simulink library "carnotUIBK"  (R2024b)
settings: Solver=VariableStepAuto  StartTime=0.0  StopTime=10.0  RelTol=1e-3  EnableMultiTasking=on
values from neighbouring files (symbols this model uses):
  area = area + room(kk).area    [THERMALZONE.m]
  boundary = BOUNDARY()    [BUILDING.m]
  building = obj    [BUILDING.m]
  C = zeros(1,length(d)+1)    [CONSTRUCTION.m]
  cp = str2num(value)    [CONSTRUCTION.m]
  pos = find(d_layer>0)    [CONSTRUCTION.m]
  rho = str2num(value)    [CONSTRUCTION.m]
  type = 1    [CONSTRUCTION.m]
  zone = obj.zone(ind)    [THERMALZONE.m]
undefined symbols (not defined in the file or in its folder): A, amb_factor, B, const, control, Dd, get_building, height, p, Qdot_C, Qdot_H, Qdot_I_electricity, Qdot_I_light, Qdot_I_person, Qdot_S, Qdot_T_ground, Qdot_T_neighbour, Qdot_T_opaque, Qdot_T_window, Qdot_V_infiltration, Qdot_V_mech, Qdot_V_window, r_frame, solar_ratio, solar_ratio1, solar_ratio2, Tc, Tr, Ts, Uvalue, view_factor, wall, wallsurface, window, window_height, window_heigth, window_width, windowsurface, x_CO2, x_H2O, x_VOC, z
libraries: carnot x105, $bdroot x22, simulink x18, simulink_extras x14
(part 4 of 13)

== system carnotUIBK/wall_intersection/EMPTY ==
  AIB1 : Inport
  AIB2 : Inport  Port=2
  Qdot_sol1 : Inport  Port=3
  Qdot_sol2 : Inport  Port=4
  Constant : Constant  Value=zeros(1,2)
  Constant1 : Constant  Value=zeros(1,5)
  Constant2 : Constant  Value=zeros(1,12)
  Constant3 : Constant  Value=zeros(1,2)
  Constant4 : Constant  Value=zeros(1,5)
  Constant5 : Constant  Value=zeros(1,12)
  Mux1 : Mux  Inputs=[2 5 12]
  Mux2 : Mux  Inputs=[2 5 12]
  Terminator{,2,4..5} (4 alike) : Terminator
  solar_ratio1 : Gain  Gain=solar_ratio1
  solar_ratio2 : Gain  Gain=solar_ratio2
  "[S1]" : Outport  VectorParamsAs1DForOutWhenUnconnected=off
  "[S2]" : Outport  Port=2  VectorParamsAs1DForOutWhenUnconnected=off
  wires:
  solar_ratio1/1 -> Terminator4/1
  Constant2/1 -> Mux1/3
  Qdot_sol1/1 -> solar_ratio1/1
  AIB1/1 -> Terminator2/1
  Constant/1 -> Mux1/1
  Mux1/1 -> "[S1]"/1
  Constant1/1 -> Mux1/2
  AIB2/1 -> Terminator/1
  solar_ratio2/1 -> Terminator5/1
  Qdot_sol2/1 -> solar_ratio2/1
  Constant5/1 -> Mux2/3
  Constant3/1 -> Mux2/1
  Mux2/1 -> "[S2]"/1
  Constant4/1 -> Mux2/2

== system carnotUIBK/wall_intersection/R-C model ==
  AIB1 : Inport
  AIB2 : Inport  Port=2
  Qdot_sol1 : Inport  Port=3
  Qdot_sol2 : Inport  Port=4
  Ground : Ground
  Terminator{,1..3,5} (5 alike) : Terminator
  Wall_basic1 : carnot/Basic/Thermal_Models/Wall_basic  tau=tau  t0=t0  d=d  dactive=dactive  cond=cond  cwall=cwall  rho=rho
      settings: SourceProductName=Carnot
  alpha_i1 : Subsystem  Variant=on  mask{view_factor=view_factor}
  alpha_i2 : Subsystem  Variant=on  mask{view_factor=amb_factor}
  nohygrothermal : Constant  Value=0
  solar_ratio1 : Gain  Gain=solar_ratio1
  solar_ratio2 : Gain  Gain=solar_ratio2
  "[S1]" : Outport  VectorParamsAs1DForOutWhenUnconnected=off
  "[S2]" : Outport  Port=2  VectorParamsAs1DForOutWhenUnconnected=off
  wires:
  alpha_i1/2("[S]") -> "[S1]"/1
  alpha_i1/3(alpha_c) -> Terminator/1
  nohygrothermal/1 -> alpha_i2/4(phis), alpha_i1/4(phis)
  solar_ratio1/1 -> alpha_i1/3(Qdot sol)
  Qdot_sol1/1 -> solar_ratio1/1
  alpha_i1/1(qdots) -> Wall_basic1/3
  alpha_i2/1(qdots) -> Wall_basic1/1
  Wall_basic1/3 -> alpha_i1/1(Ts)
  Wall_basic1/1 -> alpha_i2/1(Ts)
  Wall_basic1/2 -> Terminator5/1
  Ground/1 -> Wall_basic1/2
  Qdot_sol2/1 -> solar_ratio2/1
  AIB1/1 -> alpha_i1/2(AIB)
  AIB2/1 -> alpha_i2/2(AIB)
  solar_ratio2/1 -> alpha_i2/3(Qdot sol)
  alpha_i2/3(alpha_c) -> Terminator2/1
  alpha_i2/2("[S]") -> "[S2]"/1
  alpha_i1/4(phi_i_1/100) -> Terminator1/1
  alpha_i2/4(phi_i_1/100) -> Terminator3/1

== system carnotUIBK/wall_intersection/UA ==
  AIB1 : Inport
  AIB2 : Inport  Port=2
  Qdot_sol1 : Inport  Port=3
  Qdot_sol2 : Inport  Port=4
  1/U : Constant  Value=1/U
  Add : Sum  Inputs=2
  Add1 : Sum  Inputs=+-
  Bus Selector1 : BusSelector  OutputSignals=Ts
  Bus Selector2 : BusSelector  OutputSignals=Ts
  Constant1 : Constant  Value=zeros(1,9)
  Constant10 : Constant  Value=zeros(1,9)
  Constant2 : Constant  Value=zeros(1,7)
  Constant8 : Constant  Value=zeros(1,7)
  Gain : Gain  Gain=-1
  Mux1 : Mux  Inputs=[1 1 7 1 9]
  Mux4 : Mux  Inputs=[1 1 7 1 9]
  Qdot : Sum  Inputs=2
  Qdot1 : Sum  Inputs=2
  Qdot_T : Product  Inputs=**/
  Qdotr/Qdotc : Gain  Gain=0.5
  Qdotr/Qdotc1 : Gain  Gain=0.5
  Rsi : Subsystem  Variant=on
  solar_ratio1 : Gain  Gain=solar_ratio1
  solar_ratio2 : Gain  Gain=solar_ratio2
  wallsurface : Constant  Value=wallsurface
  "[S1]" : Outport  VectorParamsAs1DForOutWhenUnconnected=off
  "[S2]" : Outport  Port=2  VectorParamsAs1DForOutWhenUnconnected=off
  wires:
  Qdot_sol1/1 -> solar_ratio1/1
  Qdot_sol2/1 -> solar_ratio2/1
  Bus Selector1/1 -> Add1/2  "<Ts>"
  Add1/1 -> Qdot_T/1
  Add/1 -> Qdot_T/3
  wallsurface/1 -> Qdot_T/2
  Rsi/1(Rsi) -> Add/2
  1/U/1 -> Add/1
  AIB1/1 -> Bus Selector1/1
  AIB2/1 -> Bus Selector2/1
  Bus Selector2/1 -> Add1/1  "<Ts>"
  Mux4/1 -> "[S1]"/1
  Qdotr/Qdotc/1 -> Mux4/2, Mux4/1
  solar_ratio1/1 -> Qdot/2
  Mux1/1 -> "[S2]"/1
  Qdotr/Qdotc1/1 -> Mux1/2, Mux1/1
  Qdot1/1 -> Mux1/4, Qdotr/Qdotc1/1
  Gain/1 -> Qdot1/1
  solar_ratio2/1 -> Qdot1/2
  Constant10/1 -> Mux4/5
  Constant8/1 -> Mux4/3
  Qdot/1 -> Mux4/4, Qdotr/Qdotc/1
  Qdot_T/1 -> Gain/1, Qdot/1
  Constant1/1 -> Mux1/5
  Constant2/1 -> Mux1/3

== system carnotUIBK/wall_intersection/hygrothermal model ==
  AIB1 : Inport
  AIB2 : Inport  Port=2
  Qdot_sol1 : Inport  Port=3
  Qdot_sol2 : Inport  Port=4
  Bus Selector : BusSelector  OutputSignals=Tc
  Bus Selector1 : BusSelector  OutputSignals=Tc
  Constant1 : Constant  Value=0
  Constant2 : Constant  Value=0
  S-Function1 : S-Function  FunctionName=pdepesim_hygro_c_v4  Parameters=xmesh,length(xmesh),X(2:end),length(d),lambda,rho,cp,mu,ufs,FSF_u,FSF_phi,FSF_dudphi,FSF_k,K_kleff,K_u,K_kl,FSF_length,K_length,T_ini,Phi_ini,T_source,Phi_source,Tdactive,Phidactive  SFunctionDeploymentMode=off  EnableBusSupport=off
  Terminator{1..6} (6 alike) : Terminator
  alpha_i1 : Subsystem  Variant=on  mask{view_factor=view_factor}
  alpha_i2 : Subsystem  Variant=on  mask{view_factor=amb_factor}
  solar_ratio1 : Gain  Gain=solar_ratio1
  solar_ratio2 : Gain  Gain=solar_ratio2
  "[S1]" : Outport  VectorParamsAs1DForOutWhenUnconnected=off
  "[S2]" : Outport  Port=2  VectorParamsAs1DForOutWhenUnconnected=off
  wires:
  S-Function1/6 -> alpha_i1/4(phis)
  S-Function1/5 -> alpha_i2/4(phis)
  S-Function1/4 -> alpha_i1/1(Ts)
  S-Function1/3 -> alpha_i2/1(Ts)
  S-Function1/8 -> Terminator3/1
  S-Function1/7 -> Terminator4/1
  S-Function1/2 -> Terminator5/1
  S-Function1/1 -> Terminator6/1
  S-Function1/9 -> Terminator2/1
  S-Function1/10 -> Terminator1/1
  Constant1/1 -> S-Function1/10
  Constant2/1 -> S-Function1/9
  alpha_i1/3(alpha_c) -> S-Function1/8
  alpha_i2/3(alpha_c) -> S-Function1/7
  alpha_i1/4(phi_i_1/100) -> S-Function1/6
  Bus Selector/1 -> S-Function1/5  "<Tc>"
  alpha_i2/4(phi_i_1/100) -> S-Function1/4
  Bus Selector1/1 -> S-Function1/3  "<Tc>"
  alpha_i1/1(qdots) -> S-Function1/2
  alpha_i2/1(qdots) -> S-Function1/1
  solar_ratio1/1 -> alpha_i1/3(Qdot sol)
  Qdot_sol1/1 -> solar_ratio1/1
  AIB1/1 -> alpha_i1/2(AIB), Bus Selector/1
  alpha_i1/2("[S]") -> "[S1]"/1
  Qdot_sol2/1 -> solar_ratio2/1
  solar_ratio2/1 -> alpha_i2/3(Qdot sol)
  AIB2/1 -> Bus Selector1/1, alpha_i2/2(AIB)
  alpha_i2/2("[S]") -> "[S2]"/1

== system carnotUIBK/wall_zone/EMPTY ==
  WDB : Inport
  GDB : Inport  Port=2
  NDB : Inport  Port=3
  AIB : Inport  Port=4
  Qdot_in : Inport  Port=5
  Qdot_sol : Inport  Port=6
  Constant : Constant  Value=zeros(1,2)
  Constant1 : Constant  Value=zeros(1,5)
  Constant2 : Constant  Value=zeros(1,12)
  Ground3 : Ground
  Mux1 : Mux  Inputs=[2 5 12]
  Terminator{,1..5} (6 alike) : Terminator
  solar_ratio : Gain  Gain=solar_ratio
  "[S]" : Outport  VectorParamsAs1DForOutWhenUnconnected=off
  theta_out : Outport  Port=2  VectorParamsAs1DForOutWhenUnconnected=off
  wires:
  NDB/1 -> Terminator1/1
  GDB/1 -> Terminator/1
  Constant1/1 -> Mux1/2
  Mux1/1 -> "[S]"/1
  Constant/1 -> Mux1/1
  Ground3/1 -> theta_out/1
  WDB/1 -> Terminator2/1
  AIB/1 -> Terminator3/1
  Qdot_sol/1 -> solar_ratio/1
  Qdot_in/1 -> Terminator5/1
  Constant2/1 -> Mux1/3
  solar_ratio/1 -> Terminator4/1

== system carnotUIBK/wall_zone/R-C model ==
  WDB : Inport
  GDB : Inport  Port=2
  NDB : Inport  Port=3
  AIB : Inport  Port=4
  Qdot_in : Inport  Port=5
  Qdot_sol : Inport  Port=6
  Bus to Vector : BusToVector
  Bus to Vector1 : BusToVector
  Constant : Constant  Value=zeros(1,17)
  Constant1 : Constant  Value=0
  Mux1 : Mux  Inputs=[17 1 1]
  Selector1 : Selector  InputPortWidth=6  IndexOptions=Index vector (dialog)  Indices=[boundary]  OutputSizes=1
  Selector2 : Selector  InputPortWidth=6  IndexOptions=Index vector (dialog)  Indices=[boundary]  OutputSizes=1
  Selector4 : Selector  InputPortWidth=NUMBEROFWINDOWSINZONESANDINTERSECTIONS  IndexOptions=Index vector (dialog)  Indices=[wall]  OutputSizes=1
  Terminator{,1..4} (5 alike) : Terminator
  Wall_basic : carnot/Basic/Thermal_Models/Wall_basic  tau=tau  t0=t0  d=d  dactive=dactive  cond=cond  cwall=cwall  rho=rho
      settings: SourceProductName=Carnot
  alpha_e : Subsystem  Variant=on
  alpha_i : Subsystem  Variant=on  mask{view_factor=view_factor}
  nohygrothermal : Constant  Value=0
  per surface : Gain  Gain=1/wallsurface  SaturateOnIntegerOverflow=on  OutDataTypeStr=Inherit: Same as input  ParamDataTypeStr=Inherit: Same as input
  solar_ratio : Gain  Gain=solar_ratio
  sum[S] : Sum  Inputs=3
  "[S]" : Outport  VectorParamsAs1DForOutWhenUnconnected=off
  theta_out : Outport  Port=2  VectorParamsAs1DForOutWhenUnconnected=off
  wires:
  per surface/1 -> Wall_basic/2
  Wall_basic/2 -> theta_out/1
  WDB/1 -> alpha_e/1(WDB)
  Qdot_in/1 -> Selector4/1
  Wall_basic/1 -> alpha_e/5(Ts)
  Wall_basic/3 -> alpha_i/1(Ts)
  AIB/1 -> alpha_i/2(AIB), alpha_e/4(AIB)
  alpha_e/1(qdots) -> Wall_basic/1
  alpha_i/1(qdots) -> Wall_basic/3
  Qdot_sol/1 -> solar_ratio/1
  Selector4/1 -> Mux1/2, per surface/1
  Bus to Vector/1 -> Selector1/1
  Bus to Vector1/1 -> Selector2/1
  GDB/1 -> Bus to Vector/1
  NDB/1 -> Bus to Vector1/1
  solar_ratio/1 -> alpha_i/3(Qdot sol), alpha_e/6(Qdot_sol)
  nohygrothermal/1 -> alpha_i/4(phis), alpha_e/7(phis)
  alpha_i/3(alpha_c) -> Terminator/1
  alpha_i/4(phi_i_1/100) -> Terminator1/1
  alpha_i/2("[S]") -> sum[S]/2
  sum[S]/1 -> "[S]"/1
  Selector1/1 -> alpha_e/2(GDB)
  Selector2/1 -> alpha_e/3(NDB)
  alpha_e/2("[S]") -> sum[S]/1
  alpha_e/3(alpha_c) -> Terminator2/1
  alpha_e/4(phi_e_1/100) -> Terminator3/1
  Constant/1 -> Mux1/1
  Constant1/1 -> Mux1/3
  Mux1/1 -> sum[S]/3
  alpha_e/5(theta_e) -> Terminator4/1

== system carnotUIBK/wall_zone/UA ==
  WDB : Inport
  GDB : Inport  Port=2
  NDB : Inport  Port=3
  AIB : Inport  Port=4
  Qdot_in : Inport  Port=5
  Qdot_sol : Inport  Port=6
  1/U : Constant  Value=1/U
  Bus to Vector : BusToVector
  Bus to Vector1 : BusToVector
  Ground : Ground
  Rse : Subsystem  Variant=on
  Rsi : Subsystem  Variant=on
  Selector : Selector  InputPortWidth=6  IndexOptions=Index vector (dialog)  Indices=[boundary]  OutputSizes=1
  Selector1 : Selector  InputPortWidth=6  IndexOptions=Index vector (dialog)  Indices=[boundary]  OutputSizes=1
  Selector2 : Selector  InputPortWidth=NUMBEROFWINDOWSINZONESANDINTERSECTIONS  IndexOptions=Index vector (dialog)  Indices=[wall]  OutputSizes=1
  solar_ratio : Gain  Gain=solar_ratio
  "[S]" : Outport  VectorParamsAs1DForOutWhenUnconnected=off
  theta_out : Outport  Port=2  VectorParamsAs1DForOutWhenUnconnected=off
  wires:
  NDB/1 -> Bus to Vector1/1
  GDB/1 -> Bus to Vector/1
  WDB/1 -> Rse/1(WDB)
  Rse/1("[S]") -> "[S]"/1
  Ground/1 -> theta_out/1
  AIB/1 -> Rse/4(AIB)
  Qdot_sol/1 -> solar_ratio/1
  1/U/1 -> Rse/7(R)
  Rsi/1(Rsi) -> Rse/8(Rsi)
  Qdot_in/1 -> Selector2/1
  Bus to Vector/1 -> Selector/1
  Bus to Vector1/1 -> Selector1/1
  Selector/1 -> Rse/2(GDB)
  Selector1/1 -> Rse/3(NDB)
  Selector2/1 -> Rse/6(Qdot_in)
  solar_ratio/1 -> Rse/5(Qdot_sol)

== system carnotUIBK/wall_zone/hygrothermal model ==
  WDB : Inport
  GDB : Inport  Port=2
  NDB : Inport  Port=3
  AIB : Inport  Port=4
  Qdot_in : Inport  Port=5
  Qdot_sol : Inport  Port=6
  Bus Selector : BusSelector  OutputSignals=Tc
  Bus to Vector : BusToVector
  Bus to Vector1 : BusToVector
  Constant1 : Constant  Value=0
  Constant2 : Constant  Value=0
  Ground1 : Ground
  Ground3 : Ground
  Mux1 : Mux  Inputs=[17 1 1]
  S-Function1 : S-Function  FunctionName=pdepesim_hygro_c_v4  Parameters=xmesh,length(xmesh),X(2:end),length(d),lambda,rho,cp,mu,ufs,FSF_u,FSF_phi,FSF_dudphi,FSF_k,K_kleff,K_u,K_kl,FSF_length,K_length,T_ini,Phi_ini,T_source,Phi_source,Tdactive,Phidactive  SFunctionDeploymentMode=off  EnableBusSupport=off
  Selector1 : Selector  InputPortWidth=6  IndexOptions=Index vector (dialog)  Indices=[boundary]  OutputSizes=1
  Selector2 : Selector  InputPortWidth=6  IndexOptions=Index vector (dialog)  Indices=[boundary]  OutputSizes=1
  Selector4 : Selector  InputPortWidth=NUMBEROFWINDOWSINZONESANDINTERSECTIONS  IndexOptions=Index vector (dialog)  Indices=[wall]  OutputSizes=1
  Terminator{,1..6} (7 alike) : Terminator
  alpha_e : Subsystem  Variant=on
  alpha_i : Subsystem  Variant=on  mask{view_factor=view_factor}
  per surface : Gain  Gain=1/wallsurface  SaturateOnIntegerOverflow=on  OutDataTypeStr=Inherit: Same as input  ParamDataTypeStr=Inherit: Same as input
  solar_ratio : Gain  Gain=solar_ratio
  sum[S] : Sum  Inputs=3
  "[S]" : Outport  VectorParamsAs1DForOutWhenUnconnected=off
  theta_out : Outport  Port=2  VectorParamsAs1DForOutWhenUnconnected=off
  wires:
  WDB/1 -> alpha_e/1(WDB)
  Qdot_in/1 -> Selector4/1
  AIB/1 -> alpha_e/4(AIB), Bus Selector/1, alpha_i/2(AIB)
  Qdot_sol/1 -> solar_ratio/1
  Selector4/1 -> Mux1/2, per surface/1
  Bus to Vector/1 -> Selector1/1
  Bus to Vector1/1 -> Selector2/1
  GDB/1 -> Bus to Vector/1
  NDB/1 -> Bus to Vector1/1
  solar_ratio/1 -> alpha_e/6(Qdot_sol), alpha_i/3(Qdot sol)
  alpha_i/2("[S]") -> sum[S]/2
  sum[S]/1 -> "[S]"/1
  Selector1/1 -> alpha_e/2(GDB)
  Selector2/1 -> alpha_e/3(NDB)
  alpha_e/2("[S]") -> sum[S]/1
  Ground3/1 -> Mux1/1
  Ground1/1 -> Mux1/3
  Mux1/1 -> sum[S]/3
  alpha_e/1(qdots) -> S-Function1/1
  alpha_i/1(qdots) -> S-Function1/2
  alpha_e/5(theta_e) -> S-Function1/3
  alpha_e/4(phi_e_1/100) -> S-Function1/4
  Bus Selector/1 -> S-Function1/5  "<Tc>"
  alpha_i/4(phi_i_1/100) -> S-Function1/6
  alpha_e/3(alpha_c) -> S-Function1/7
  alpha_i/3(alpha_c) -> S-Function1/8
  per surface/1 -> Terminator/1
  Constant2/1 -> S-Function1/9
  Constant1/1 -> S-Function1/10
  S-Function1/10 -> Terminator1/1
  S-Function1/9 -> Terminator2/1
  S-Function1/1 -> Terminator6/1
  S-Function1/2 -> Terminator5/1
  S-Function1/7 -> Terminator4/1
  S-Function1/8 -> Terminator3/1
  S-Function1/3 -> alpha_e/5(Ts)
  S-Function1/4 -> alpha_i/1(Ts)
  S-Function1/5 -> alpha_e/7(phis)
  S-Function1/6 -> alpha_i/4(phis)

== system carnotUIBK/window/EMTPY ==
  WDB : Inport
  AIB : Inport  Port=2
  control : Inport  Port=3
  Constant : Constant  Value=zeros(1,2)
  Constant1 : Constant  Value=zeros(1,5)
  Constant2 : Constant  Value=zeros(1,12)
  Mux1 : Mux  Inputs=[2 5 12]
  Selector1 : Selector  InputPortWidth=NUMBEROFCONTROLS  IndexOptions=Index vector (dialog)  Indices=[control]  OutputSizes=1
  Terminator1 : Terminator
  Terminator2 : Terminator
  Terminator4 : Terminator
  "[S]" : Outport  VectorParamsAs1DForOutWhenUnconnected=off
  wires:
  Constant2/1 -> Mux1/3
  Constant/1 -> Mux1/1
  Mux1/1 -> "[S]"/1
  Constant1/1 -> Mux1/2
  control/1 -> Selector1/1
  AIB/1 -> Terminator1/1
  WDB/1 -> Terminator2/1
  Selector1/1 -> Terminator4/1

== system carnotUIBK/window/window_CARNOT ==
  WDB : Inport
  AIB : Inport  Port=2
  control : Inport  Port=3
  Add : Sum  Inputs=+-
  Constant : Constant
  Product : Product
  Selector1 : Selector  InputPortWidth=NUMBEROFCONTROLS  IndexOptions=Index vector (dialog)  Indices=[control]  OutputSizes=1
  Terminator1 : Terminator
  Wall_basic : carnot/Basic/Thermal_Models/Wall_basic  tau=3600  t0=20  d=[0.1 0.1 0.1]  dactive=-1  cond=[1 2 1]  cwall=[800 1000 800]  rho=[2000 2700 2000]
      settings: SourceProductName=Carnot
  alfa_window_in : Subsystem  mask(ALFA){}
      mask help:
      | Convective and radiative heat transfer at the INDOOR SURFACE OF A VERTICAL WINDOW with 1-4 layers (each 3 ... 8 mm thick).
      |
      | Ts  : temperature of window surface, °C,
      | [sun_t]  : sun data (incidence angle, direct and diffuse radiation
      |     at tilted window surface),
      | [AIV]  : conditions of zone node,
      | qdots  : specific heat flow into window construction, W/m^2,
      | qdot_abs : specific irradiation absorption within window
      |     construction,  W/m^2,
      | [S]  : heat and air flow to zone node.
  alfa_window_out : Subsystem  mask(ALFA){}
      mask help:
      | Convective and radiative heat transfer at the OUTDOOR SURFACE OF A VERTICAL WINDOW.
      |
      | [W*] : modified weather data, adapted to height over ground,
      | Ts : temperature of outdoor window surface, °C,
      | qdots : specific heat flow into window construction, W/m^2,
      | [sun_t] : sun data (incidence angle, direct and diffuse radiation
      |                  at tilted window surface).
  position1 : Constant
  sum[S] : Sum  Inputs=2
  "[S]" : Outport  VectorParamsAs1DForOutWhenUnconnected=off
  wires:
  Wall_basic/1 -> alfa_window_out/3(Ts1)
  AIB/1 -> alfa_window_in/3("[AIV]")
  alfa_window_in/1(qdots2) -> Wall_basic/3
  WDB/1 -> alfa_window_out/1(WDB)
  alfa_window_out/1("[sun_t]") -> alfa_window_in/2("[sun_t]")
  Wall_basic/2 -> Terminator1/1
  alfa_window_out/2(qdots1) -> Wall_basic/1
  Wall_basic/3 -> alfa_window_in/1(Ts2)
  alfa_window_in/2(qdot_abs) -> Wall_basic/2
  position1/1 -> Product/1
  Product/1 -> alfa_window_out/2(g)
  control/1 -> Selector1/1
  Add/1 -> Product/2
  Constant/1 -> Add/1
  alfa_window_in/3("[S]") -> sum[S]/2
  sum[S]/1 -> "[S]"/1
  alfa_window_out/3("[S]") -> sum[S]/1
  Selector1/1 -> Add/2

== system carnotUIBK/window/window_TF ==
  WDB : Inport
  AIB : Inport  Port=2
  control : Inport  Port=3
  Add : Sum  Inputs=+-
  Constant : Constant
  Constant1 : Constant  Value=0
  Product : Product  Inputs=4
  Selector1 : Selector  InputPortWidth=NUMBEROFCONTROLS  IndexOptions=Index vector (dialog)  Indices=[control]  OutputSizes=1
  alfa_window_in : Subsystem  mask(ALFA){}
      mask help:
      | Convective and radiative heat transfer at the INDOOR SURFACE OF A VERTICAL WINDOW with 1-4 layers (each 3 ... 8 mm thick).
      |
      | Ts  : temperature of window surface, °C,
      | [sun_t]  : sun data (incidence angle, direct and diffuse radiation
      |     at tilted window surface),
      | [AIV]  : conditions of zone node,
      | qdots  : specific heat flow into window construction, W/m^2,
      | [S]  : heat and air flow to zone node.
  alfa_window_out : Subsystem  mask(ALFA){}
      mask help:
      | Convective and radiative heat transfer at the OUTDOOR SURFACE OF A VERTICAL WINDOW.
      |
      | [W*] : modified weather data, adapted to height over ground,
      | Ts : temperature of outdoor window surface, °C,
      | qdots : specific heat flow into window construction, W/m^2,
      | [sun_t] : sun data (incidence angle, direct and diffuse radiation
      |                  at tilted window surface).
  lambda_window : Subsystem  mask(LAMBDA){}
      mask help:
      | Heat conduction through a transparent component (window).
      |
      | qdots1	: specific heat flow vertical on surface 1, W/m²
      | qdots2	: specific heat flow vertical on surface 2, W/m²
      | Ts1	: temperature of surface 1, °C
      | Ts2	: temperature of surface 2, °C
      |
      | NOTE CONVENTION for INPUT NUMBER:
      | "1"	  indoor surface of an outer window OR
      | 	  surface "a" of an inner window OR
      |  	  surface "f" of a glass floor
      |
      | "2"	  outdoor surface of a window OR
      | 	  surface "b" of an inner window OR
      |  	  surface "c" of a glass ceiling
  position1 : Constant  Value=zone{window,15}
  position2 : Constant
  sum[S] : Sum  Inputs=2
  time_value : FromWorkspace  VariableName=z.win_factor_seq{window}
  "[S]" : Outport  VectorParamsAs1DForOutWhenUnconnected=off
  wires:
  alfa_window_out/1("[sun_t]") -> alfa_window_in/2("[sun_t]")
  alfa_window_out/2(qdots1) -> lambda_window/1(qdots1)
  alfa_window_in/1(qdots2) -> lambda_window/2(qdots2)
  AIB/1 -> alfa_window_in/3("[AIV]")
  WDB/1 -> alfa_window_out/1(WDB), alfa_window_in/4(WDB)
  sum[S]/1 -> "[S]"/1
  alfa_window_in/2("[S]") -> sum[S]/2
  alfa_window_out/3("[S]") -> sum[S]/1
  lambda_window/1(Ts1) -> alfa_window_out/3(Ts1)
  lambda_window/2(Ts2) -> alfa_window_in/1(Ts2)
  position2/1 -> Product/3
  control/1 -> Selector1/1
  Add/1 -> Product/4
  Constant/1 -> Add/1
  Product/1 -> alfa_window_out/2(g)
  Constant1/1 -> alfa_window_in/5(control)
  Selector1/1 -> Add/2
  time_value/1 -> Product/2
  position1/1 -> Product/1

== system carnotUIBK/window/window_TF_shading ==
  WDB : Inport
  AIB : Inport  Port=2
  control : Inport  Port=3
  Product : Product  Inputs=3
  Selector1 : Selector  InputPortWidth=NUMBEROFCONTROLS  IndexOptions=Index vector (dialog)  Indices=[control]  OutputSizes=1
  alfa_window_in : Subsystem  mask(ALFA){}
      mask help:
      | Convective and radiative heat transfer at the INDOOR SURFACE OF A VERTICAL WINDOW with 1-4 layers (each 3 ... 8 mm thick).
      |
      | Ts  : temperature of window surface, °C,
      | [sun_t]  : sun data (incidence angle, direct and diffuse radiation
      |     at tilted window surface),
      | [AIV]  : conditions of zone node,
      | qdots  : specific heat flow into window construction, W/m^2,
      | [S]  : heat and air flow to zone node.
  alfa_window_out : Subsystem  mask(ALFA){}
      mask help:
      | Convective and radiative heat transfer at the OUTDOOR SURFACE OF A VERTICAL WINDOW.
      |
      | [W*] : modified weather data, adapted to height over ground,
      | Ts : temperature of outdoor window surface, °C,
      | qdots : specific heat flow into window construction, W/m^2,
      | [sun_t] : sun data (incidence angle, direct and diffuse radiation
      |                  at tilted window surface).
  lambda_window : Subsystem  mask(LAMBDA){}
      mask help:
      | Heat conduction through a transparent component (window).
      |
      | qdots1	: specific heat flow vertical on surface 1, W/m²
      | qdots2	: specific heat flow vertical on surface 2, W/m²
      | Ts1	: temperature of surface 1, °C
      | Ts2	: temperature of surface 2, °C
      |
      | NOTE CONVENTION for INPUT NUMBER:
      | "1"	  indoor surface of an outer window OR
      | 	  surface "a" of an inner window OR
      |  	  surface "f" of a glass floor
      |
      | "2"	  outdoor surface of a window OR
      | 	  surface "b" of an inner window OR
      |  	  surface "c" of a glass ceiling
  position1 : Constant
  position2 : Constant  Value=zone{window,15}
  sum[S] : Sum  Inputs=2
  time_value : FromWorkspace  VariableName=z.win_factor_seq{window}
  "[S]" : Outport  VectorParamsAs1DForOutWhenUnconnected=off
  wires:
  position1/1 -> Product/3
  control/1 -> Selector1/1
  alfa_window_out/1("[sun_t]") -> alfa_window_in/2("[sun_t]")
  alfa_window_out/2(qdots1) -> lambda_window/1(qdots1)
  alfa_window_in/1(qdots2) -> lambda_window/2(qdots2)
  AIB/1 -> alfa_window_in/3("[AIV]")
  WDB/1 -> alfa_window_in/4(WDB), alfa_window_out/1(WDB)
  sum[S]/1 -> "[S]"/1
  alfa_window_in/2("[S]") -> sum[S]/2
  alfa_window_out/3("[S]") -> sum[S]/1
  lambda_window/1(Ts1) -> alfa_window_out/3(Ts1)
  lambda_window/2(Ts2) -> alfa_window_in/1(Ts2)
  Selector1/1 -> alfa_window_in/5(control)
  time_value/1 -> Product/2
  position2/1 -> Product/1
  Product/1 -> alfa_window_out/2(g)

== system carnotUIBK/HVAC/HVAC_1001_electrical heaters/electrical heater zone 1 ==
  temperature setpoint : Inport
  temperature room : Inport  Port=2
  Enable : EnablePort
  " " : Constant  Value=0
  "   " : Constant  Value=zeros(1,15)
  Bus Creator1 : BusCreator  Inputs=2
  Bus Selector5 : BusSelector  OutputSignals=Ts
  Integrator : Integrator
  Mux1 : Mux  Inputs=[1 1 15 1 1]
  PID : simulink/Continuous/PID Controller  Controller=PI  Form=Ideal  TimeDomain=Continuous-time  SampleTime=-1  IntegratorMethod=Forward Euler  ControllerParametersSource=internal  P=Kp  I=1/(Tn*60)  D=0  N=100  UseFilter=on  TunerSelectOption=Transfer Function Based (PID Tuner App)  InitialConditionSource=internal  InitialConditionForIntegrator=0  InitialConditionForFilter=0  DifferentiatorICPrevScaledInput=0  ExternalReset=none  TrackingMode=off  Kt=1  LimitOutput=on  UpperSaturationLimit=1  LowerSaturationLimit=0  LinearizeAsGain=off  AntiWindupMode=clamping  Kb=1  POutMin=[]  POutMax=[]  IOutMin=[]  IOutMax=[]  DOutMin=[]  DOutMax=[]  NOutMin=[]  NOutMax=[]  SumOutMin=[]  SumOutMax=[]  SaturationOutMin=[]  SaturationOutMax=[]  PParamMin=[]  PParamMax=[]  IParamMin=[]  IParamMax=[]  DParamMin=[]  DParamMax=[]  NParamMin=[]  NParamMax=[]  KbParamMin=[]  KbParamMax=[]  KtParamMin=[]  KtParamMax=[]  KbOutMin=[]  KbOutMax=[]  KtOutMin=[]  KtOutMax=[]  IntegratorOutMin=[]  IntegratorOutMax=[]  FilterOutMin=[]  FilterOutMax=[]  SumI1OutMin=[]  SumI1OutMax=[]  SumI2OutMin=[]  SumI2OutMax=[]  SumI3OutMin=[]  SumI3OutMax=[]  SumI4OutMin=[]  SumI4OutMax=[]  SumDOutMin=[]  SumDOutMax=[]  DifferentiatorOutMin=[]  DifferentiatorOutMax=[]  FilterDiffOutCoefMin=[]  FilterDiffOutCoefMax=[]  ReciprocalOutMin=[]  ReciprocalOutMax=[]  SumDenOutMin=[]  SumDenOutMax=[]  SumNumOutMin=[]  SumNumOutMax=[]  DivideOutMin=[]  DivideOutMax=[]  IntegratorContinuousStateAttributes=''  IntegratorStateMustResolveToSignalObject=off  IntegratorRTWStateStorageClass=Auto  FilterContinuousStateAttributes=''  FilterStateMustResolveToSignalObject=off  FilterRTWStateStorageClass=Auto  ParallelPVariant=Passthrough  IdealPVariant=InternalParameters  IVariant=InternalParameters  DVariant=Disabled  IntegratorVariant=Continuous  SatVariant=Enabled  AWVariant=ContClampingIdeal  PCopyVariant=InternalParamsIdeal  TRVariant=Disabled  FdbkBlocksVariant=Forward  IdealPFdbkVariant=Disabled  SatFdbkVariant=Disabled  DerivativeFilterVariant=Disabled  NVariant=Disabled  NCopyVariant=Disabled_SignalSpec  FilterICVariant=Disabled  IntegratorICVariant=InternalICs  ExternalResetVariant=Disabled  TRSumVariant=Passthrough  SumFdbkVariant=Disabled  SumVariant=Sum_PI
  Product : Product
  Sum13 : Sum  Inputs=|+-
  Transfer Fcn (with initial states) : Subsystem  mask(Transfer Function with Initial States){N=[1], D=[timeconst 1], X0=0}
      mask prompts: N "Numerator:"; D "Denominator:"; X0 "Initial conditions:"
      mask help: Vector expressions for numerator, and denominator. Coefficients are in descending powers of s.
      mask init:
      | [A,B,C,Dd]=tf2ss(N,D);if (isempty(X0));[m,n]=size(A);X0=zeros(1,m); end;
      mask Help: Specify the initial states for the transfer function.  The state ordering is determined by the m-file tf2ss.  There is no unique mapping of the states in a transfer function to states in a state-space representation.  However, tf2ss will consistently use the same mapping for a given transfer function.
      mask Display: dpoly(N,D,'s')
  convective : Gain  Gain=s_conv  SaturateOnIntegerOverflow=on  OutDataTypeStr=Inherit: Same as input  ParamDataTypeStr=Inherit: Same as input
  maximal power : Constant  Value=max_power
  radiative : Gain  Gain=1-s_conv  SaturateOnIntegerOverflow=on  OutDataTypeStr=Inherit: Same as input  ParamDataTypeStr=Inherit: Same as input
  "[S]" : Outport  VectorParamsAs1DForOutWhenUnconnected=off
  "[HVAC]" : Outport  Port=2  VectorParamsAs1DForOutWhenUnconnected=off
  wires:
  Sum13/1 -> PID/1
  Transfer Fcn (with initial states)/1(Out1) -> Product/1
  " "/1 -> Mux1/5
  Mux1/1 -> "[S]"/1
  convective/1 -> Mux1/1
  PID/1 -> Transfer Fcn (with initial states)/1(In1)
  maximal power/1 -> Product/2
  temperature room/1 -> Bus Selector5/1
  radiative/1 -> Mux1/2
  "   "/1 -> Mux1/3
  Product/1 -> convective/1, radiative/1, Bus Creator1/1, Integrator/1, Mux1/4  "heating power"
  Bus Selector5/1 -> Sum13/2  "<Ts>"
  temperature setpoint/1 -> Sum13/1
  Integrator/1 -> Bus Creator1/2  "heating energy"
  Bus Creator1/1 -> "[HVAC]"/1

== system carnotUIBK/HVAC/HVAC_1001_electrical heaters/electrical heater zone 10 ==
  temperature setpoint : Inport
  temperature room : Inport  Port=2
  Enable : EnablePort
  " " : Constant  Value=0
  "   " : Constant  Value=zeros(1,15)
  Bus Creator1 : BusCreator  Inputs=2
  Bus Selector5 : BusSelector  OutputSignals=Ts
  Integrator : Integrator
  Mux1 : Mux  Inputs=[1 1 15 1 1]
  PID : simulink/Continuous/PID Controller  Controller=PI  Form=Ideal  TimeDomain=Continuous-time  SampleTime=-1  IntegratorMethod=Forward Euler  ControllerParametersSource=internal  P=Kp  I=1/(Tn*60)  D=0  N=100  UseFilter=on  TunerSelectOption=Transfer Function Based (PID Tuner App)  InitialConditionSource=internal  InitialConditionForIntegrator=0  InitialConditionForFilter=0  DifferentiatorICPrevScaledInput=0  ExternalReset=none  TrackingMode=off  Kt=1  LimitOutput=on  UpperSaturationLimit=1  LowerSaturationLimit=0  LinearizeAsGain=off  AntiWindupMode=clamping  Kb=1  POutMin=[]  POutMax=[]  IOutMin=[]  IOutMax=[]  DOutMin=[]  DOutMax=[]  NOutMin=[]  NOutMax=[]  SumOutMin=[]  SumOutMax=[]  SaturationOutMin=[]  SaturationOutMax=[]  PParamMin=[]  PParamMax=[]  IParamMin=[]  IParamMax=[]  DParamMin=[]  DParamMax=[]  NParamMin=[]  NParamMax=[]  KbParamMin=[]  KbParamMax=[]  KtParamMin=[]  KtParamMax=[]  KbOutMin=[]  KbOutMax=[]  KtOutMin=[]  KtOutMax=[]  IntegratorOutMin=[]  IntegratorOutMax=[]  FilterOutMin=[]  FilterOutMax=[]  SumI1OutMin=[]  SumI1OutMax=[]  SumI2OutMin=[]  SumI2OutMax=[]  SumI3OutMin=[]  SumI3OutMax=[]  SumI4OutMin=[]  SumI4OutMax=[]  SumDOutMin=[]  SumDOutMax=[]  DifferentiatorOutMin=[]  DifferentiatorOutMax=[]  FilterDiffOutCoefMin=[]  FilterDiffOutCoefMax=[]  ReciprocalOutMin=[]  ReciprocalOutMax=[]  SumDenOutMin=[]  SumDenOutMax=[]  SumNumOutMin=[]  SumNumOutMax=[]  DivideOutMin=[]  DivideOutMax=[]  IntegratorContinuousStateAttributes=''  IntegratorStateMustResolveToSignalObject=off  IntegratorRTWStateStorageClass=Auto  FilterContinuousStateAttributes=''  FilterStateMustResolveToSignalObject=off  FilterRTWStateStorageClass=Auto  ParallelPVariant=Passthrough  IdealPVariant=InternalParameters  IVariant=InternalParameters  DVariant=Disabled  IntegratorVariant=Continuous  SatVariant=Enabled  AWVariant=ContClampingIdeal  PCopyVariant=InternalParamsIdeal  TRVariant=Disabled  FdbkBlocksVariant=Forward  IdealPFdbkVariant=Disabled  SatFdbkVariant=Disabled  DerivativeFilterVariant=Disabled  NVariant=Disabled  NCopyVariant=Disabled_SignalSpec  FilterICVariant=Disabled  IntegratorICVariant=InternalICs  ExternalResetVariant=Disabled  TRSumVariant=Passthrough  SumFdbkVariant=Disabled  SumVariant=Sum_PI
  Product : Product
  Sum13 : Sum  Inputs=|+-
  Transfer Fcn (with initial states) : Subsystem  mask(Transfer Function with Initial States){N=[1], D=[timeconst 1], X0=0}
      mask prompts: N "Numerator:"; D "Denominator:"; X0 "Initial conditions:"
      mask help: Vector expressions for numerator, and denominator. Coefficients are in descending powers of s.
      mask init:
      | [A,B,C,Dd]=tf2ss(N,D);if (isempty(X0));[m,n]=size(A);X0=zeros(1,m); end;
      mask Help: Specify the initial states for the transfer function.  The state ordering is determined by the m-file tf2ss.  There is no unique mapping of the states in a transfer function to states in a state-space representation.  However, tf2ss will consistently use the same mapping for a given transfer function.
      mask Display: dpoly(N,D,'s')
  convective : Gain  Gain=s_conv  SaturateOnIntegerOverflow=on  OutDataTypeStr=Inherit: Same as input  ParamDataTypeStr=Inherit: Same as input
  maximal power : Constant  Value=max_power
  radiative : Gain  Gain=1-s_conv  SaturateOnIntegerOverflow=on  OutDataTypeStr=Inherit: Same as input  ParamDataTypeStr=Inherit: Same as input
  "[S]" : Outport  VectorParamsAs1DForOutWhenUnconnected=off
  "[HVAC]" : Outport  Port=2  VectorParamsAs1DForOutWhenUnconnected=off
  wires:
  Bus Creator1/1 -> "[HVAC]"/1
  Integrator/1 -> Bus Creator1/2  "heating energy"
  temperature setpoint/1 -> Sum13/1
  Bus Selector5/1 -> Sum13/2  "<Ts>"
  Product/1 -> Mux1/4, Integrator/1, Bus Creator1/1, radiative/1, convective/1  "heating power"
  "   "/1 -> Mux1/3
  radiative/1 -> Mux1/2
  temperature room/1 -> Bus Selector5/1
  maximal power/1 -> Product/2
  PID/1 -> Transfer Fcn (with initial states)/1(In1)
  convective/1 -> Mux1/1
  Mux1/1 -> "[S]"/1
  " "/1 -> Mux1/5
  Transfer Fcn (with initial states)/1(Out1) -> Product/1
  Sum13/1 -> PID/1

== system carnotUIBK/HVAC/HVAC_1001_electrical heaters/electrical heater zone 2 ==
  temperature setpoint : Inport
  temperature room : Inport  Port=2
  Enable : EnablePort
  " " : Constant  Value=0
  "   " : Constant  Value=zeros(1,15)
  Bus Creator1 : BusCreator  Inputs=2
  Bus Selector5 : BusSelector  OutputSignals=Ts
  Integrator : Integrator
  Mux1 : Mux  Inputs=[1 1 15 1 1]
  PID : simulink/Continuous/PID Controller  Controller=PI  Form=Ideal  TimeDomain=Continuous-time  SampleTime=-1  IntegratorMethod=Forward Euler  ControllerParametersSource=internal  P=Kp  I=1/(Tn*60)  D=0  N=100  UseFilter=on  TunerSelectOption=Transfer Function Based (PID Tuner App)  InitialConditionSource=internal  InitialConditionForIntegrator=0  InitialConditionForFilter=0  DifferentiatorICPrevScaledInput=0  ExternalReset=none  TrackingMode=off  Kt=1  LimitOutput=on  UpperSaturationLimit=1  LowerSaturationLimit=0  LinearizeAsGain=off  AntiWindupMode=clamping  Kb=1  POutMin=[]  POutMax=[]  IOutMin=[]  IOutMax=[]  DOutMin=[]  DOutMax=[]  NOutMin=[]  NOutMax=[]  SumOutMin=[]  SumOutMax=[]  SaturationOutMin=[]  SaturationOutMax=[]  PParamMin=[]  PParamMax=[]  IParamMin=[]  IParamMax=[]  DParamMin=[]  DParamMax=[]  NParamMin=[]  NParamMax=[]  KbParamMin=[]  KbParamMax=[]  KtParamMin=[]  KtParamMax=[]  KbOutMin=[]  KbOutMax=[]  KtOutMin=[]  KtOutMax=[]  IntegratorOutMin=[]  IntegratorOutMax=[]  FilterOutMin=[]  FilterOutMax=[]  SumI1OutMin=[]  SumI1OutMax=[]  SumI2OutMin=[]  SumI2OutMax=[]  SumI3OutMin=[]  SumI3OutMax=[]  SumI4OutMin=[]  SumI4OutMax=[]  SumDOutMin=[]  SumDOutMax=[]  DifferentiatorOutMin=[]  DifferentiatorOutMax=[]  FilterDiffOutCoefMin=[]  FilterDiffOutCoefMax=[]  ReciprocalOutMin=[]  ReciprocalOutMax=[]  SumDenOutMin=[]  SumDenOutMax=[]  SumNumOutMin=[]  SumNumOutMax=[]  DivideOutMin=[]  DivideOutMax=[]  IntegratorContinuousStateAttributes=''  IntegratorStateMustResolveToSignalObject=off  IntegratorRTWStateStorageClass=Auto  FilterContinuousStateAttributes=''  FilterStateMustResolveToSignalObject=off  FilterRTWStateStorageClass=Auto  ParallelPVariant=Passthrough  IdealPVariant=InternalParameters  IVariant=InternalParameters  DVariant=Disabled  IntegratorVariant=Continuous  SatVariant=Enabled  AWVariant=ContClampingIdeal  PCopyVariant=InternalParamsIdeal  TRVariant=Disabled  FdbkBlocksVariant=Forward  IdealPFdbkVariant=Disabled  SatFdbkVariant=Disabled  DerivativeFilterVariant=Disabled  NVariant=Disabled  NCopyVariant=Disabled_SignalSpec  FilterICVariant=Disabled  IntegratorICVariant=InternalICs  ExternalResetVariant=Disabled  TRSumVariant=Passthrough  SumFdbkVariant=Disabled  SumVariant=Sum_PI
  Product : Product
  Sum13 : Sum  Inputs=|+-
  Transfer Fcn (with initial states) : Subsystem  mask(Transfer Function with Initial States){N=[1], D=[timeconst 1], X0=0}
      mask prompts: N "Numerator:"; D "Denominator:"; X0 "Initial conditions:"
      mask help: Vector expressions for numerator, and denominator. Coefficients are in descending powers of s.
      mask init:
      | [A,B,C,Dd]=tf2ss(N,D);if (isempty(X0));[m,n]=size(A);X0=zeros(1,m); end;
      mask Help: Specify the initial states for the transfer function.  The state ordering is determined by the m-file tf2ss.  There is no unique mapping of the states in a transfer function to states in a state-space representation.  However, tf2ss will consistently use the same mapping for a given transfer function.
      mask Display: dpoly(N,D,'s')
  convective : Gain  Gain=s_conv  SaturateOnIntegerOverflow=on  OutDataTypeStr=Inherit: Same as input  ParamDataTypeStr=Inherit: Same as input
  maximal power : Constant  Value=max_power
  radiative : Gain  Gain=1-s_conv  SaturateOnIntegerOverflow=on  OutDataTypeStr=Inherit: Same as input  ParamDataTypeStr=Inherit: Same as input
  "[S]" : Outport  VectorParamsAs1DForOutWhenUnconnected=off
  "[HVAC]" : Outport  Port=2  VectorParamsAs1DForOutWhenUnconnected=off
  wires:
  Bus Creator1/1 -> "[HVAC]"/1
  Integrator/1 -> Bus Creator1/2  "heating energy"
  temperature setpoint/1 -> Sum13/1
  Bus Selector5/1 -> Sum13/2  "<Ts>"
  Product/1 -> Mux1/4, Integrator/1, Bus Creator1/1, radiative/1, convective/1  "heating power"
  "   "/1 -> Mux1/3
  radiative/1 -> Mux1/2
  temperature room/1 -> Bus Selector5/1
  maximal power/1 -> Product/2
  PID/1 -> Transfer Fcn (with initial states)/1(In1)
  convective/1 -> Mux1/1
  Mux1/1 -> "[S]"/1
  " "/1 -> Mux1/5
  Transfer Fcn (with initial states)/1(Out1) -> Product/1
  Sum13/1 -> PID/1

== system carnotUIBK/HVAC/HVAC_1001_electrical heaters/electrical heater zone 3 ==
  temperature setpoint : Inport
  temperature room : Inport  Port=2
  Enable : EnablePort
  " " : Constant  Value=0
  "   " : Constant  Value=zeros(1,15)
  Bus Creator1 : BusCreator  Inputs=2
  Bus Selector5 : BusSelector  OutputSignals=Ts
  Integrator : Integrator
  Mux1 : Mux  Inputs=[1 1 15 1 1]
  PID : simulink/Continuous/PID Controller  Controller=PI  Form=Ideal  TimeDomain=Continuous-time  SampleTime=-1  IntegratorMethod=Forward Euler  ControllerParametersSource=internal  P=Kp  I=1/(Tn*60)  D=0  N=100  UseFilter=on  TunerSelectOption=Transfer Function Based (PID Tuner App)  InitialConditionSource=internal  InitialConditionForIntegrator=0  InitialConditionForFilter=0  DifferentiatorICPrevScaledInput=0  ExternalReset=none  TrackingMode=off  Kt=1  LimitOutput=on  UpperSaturationLimit=1  LowerSaturationLimit=0  LinearizeAsGain=off  AntiWindupMode=clamping  Kb=1  POutMin=[]  POutMax=[]  IOutMin=[]  IOutMax=[]  DOutMin=[]  DOutMax=[]  NOutMin=[]  NOutMax=[]  SumOutMin=[]  SumOutMax=[]  SaturationOutMin=[]  SaturationOutMax=[]  PParamMin=[]  PParamMax=[]  IParamMin=[]  IParamMax=[]  DParamMin=[]  DParamMax=[]  NParamMin=[]  NParamMax=[]  KbParamMin=[]  KbParamMax=[]  KtParamMin=[]  KtParamMax=[]  KbOutMin=[]  KbOutMax=[]  KtOutMin=[]  KtOutMax=[]  IntegratorOutMin=[]  IntegratorOutMax=[]  FilterOutMin=[]  FilterOutMax=[]  SumI1OutMin=[]  SumI1OutMax=[]  SumI2OutMin=[]  SumI2OutMax=[]  SumI3OutMin=[]  SumI3OutMax=[]  SumI4OutMin=[]  SumI4OutMax=[]  SumDOutMin=[]  SumDOutMax=[]  DifferentiatorOutMin=[]  DifferentiatorOutMax=[]  FilterDiffOutCoefMin=[]  FilterDiffOutCoefMax=[]  ReciprocalOutMin=[]  ReciprocalOutMax=[]  SumDenOutMin=[]  SumDenOutMax=[]  SumNumOutMin=[]  SumNumOutMax=[]  DivideOutMin=[]  DivideOutMax=[]  IntegratorContinuousStateAttributes=''  IntegratorStateMustResolveToSignalObject=off  IntegratorRTWStateStorageClass=Auto  FilterContinuousStateAttributes=''  FilterStateMustResolveToSignalObject=off  FilterRTWStateStorageClass=Auto  ParallelPVariant=Passthrough  IdealPVariant=InternalParameters  IVariant=InternalParameters  DVariant=Disabled  IntegratorVariant=Continuous  SatVariant=Enabled  AWVariant=ContClampingIdeal  PCopyVariant=InternalParamsIdeal  TRVariant=Disabled  FdbkBlocksVariant=Forward  IdealPFdbkVariant=Disabled  SatFdbkVariant=Disabled  DerivativeFilterVariant=Disabled  NVariant=Disabled  NCopyVariant=Disabled_SignalSpec  FilterICVariant=Disabled  IntegratorICVariant=InternalICs  ExternalResetVariant=Disabled  TRSumVariant=Passthrough  SumFdbkVariant=Disabled  SumVariant=Sum_PI
  Product : Product
  Sum13 : Sum  Inputs=|+-
  Transfer Fcn (with initial states) : Subsystem  mask(Transfer Function with Initial States){N=[1], D=[timeconst 1], X0=0}
      mask prompts: N "Numerator:"; D "Denominator:"; X0 "Initial conditions:"
      mask help: Vector expressions for numerator, and denominator. Coefficients are in descending powers of s.
      mask init:
      | [A,B,C,Dd]=tf2ss(N,D);if (isempty(X0));[m,n]=size(A);X0=zeros(1,m); end;
      mask Help: Specify the initial states for the transfer function.  The state ordering is determined by the m-file tf2ss.  There is no unique mapping of the states in a transfer function to states in a state-space representation.  However, tf2ss will consistently use the same mapping for a given transfer function.
      mask Display: dpoly(N,D,'s')
  convective : Gain  Gain=s_conv  SaturateOnIntegerOverflow=on  OutDataTypeStr=Inherit: Same as input  ParamDataTypeStr=Inherit: Same as input
  maximal power : Constant  Value=max_power
  radiative : Gain  Gain=1-s_conv  SaturateOnIntegerOverflow=on  OutDataTypeStr=Inherit: Same as input  ParamDataTypeStr=Inherit: Same as input
  "[S]" : Outport  VectorParamsAs1DForOutWhenUnconnected=off
  "[HVAC]" : Outport  Port=2  VectorParamsAs1DForOutWhenUnconnected=off
  wires:
  Sum13/1 -> PID/1
  Transfer Fcn (with initial states)/1(Out1) -> Product/1
  " "/1 -> Mux1/5
  Mux1/1 -> "[S]"/1
  convective/1 -> Mux1/1
  PID/1 -> Transfer Fcn (with initial states)/1(In1)
  maximal power/1 -> Product/2
  temperature room/1 -> Bus Selector5/1
  radiative/1 -> Mux1/2
  "   "/1 -> Mux1/3
  Product/1 -> convective/1, radiative/1, Bus Creator1/1, Integrator/1, Mux1/4  "heating power"
  Bus Selector5/1 -> Sum13/2  "<Ts>"
  temperature setpoint/1 -> Sum13/1
  Integrator/1 -> Bus Creator1/2  "heating energy"
  Bus Creator1/1 -> "[HVAC]"/1

== system carnotUIBK/HVAC/HVAC_1001_electrical heaters/electrical heater zone 4 ==
  temperature setpoint : Inport
  temperature room : Inport  Port=2
  Enable : EnablePort
  " " : Constant  Value=0
  "   " : Constant  Value=zeros(1,15)
  Bus Creator1 : BusCreator  Inputs=2
  Bus Selector5 : BusSelector  OutputSignals=Ts
  Integrator : Integrator
  Mux1 : Mux  Inputs=[1 1 15 1 1]
  PID : simulink/Continuous/PID Controller  Controller=PI  Form=Ideal  TimeDomain=Continuous-time  SampleTime=-1  IntegratorMethod=Forward Euler  ControllerParametersSource=internal  P=Kp  I=1/(Tn*60)  D=0  N=100  UseFilter=on  TunerSelectOption=Transfer Function Based (PID Tuner App)  InitialConditionSource=internal  InitialConditionForIntegrator=0  InitialConditionForFilter=0  DifferentiatorICPrevScaledInput=0  ExternalReset=none  TrackingMode=off  Kt=1  LimitOutput=on  UpperSaturationLimit=1  LowerSaturationLimit=0  LinearizeAsGain=off  AntiWindupMode=clamping  Kb=1  POutMin=[]  POutMax=[]  IOutMin=[]  IOutMax=[]  DOutMin=[]  DOutMax=[]  NOutMin=[]  NOutMax=[]  SumOutMin=[]  SumOutMax=[]  SaturationOutMin=[]  SaturationOutMax=[]  PParamMin=[]  PParamMax=[]  IParamMin=[]  IParamMax=[]  DParamMin=[]  DParamMax=[]  NParamMin=[]  NParamMax=[]  KbParamMin=[]  KbParamMax=[]  KtParamMin=[]  KtParamMax=[]  KbOutMin=[]  KbOutMax=[]  KtOutMin=[]  KtOutMax=[]  IntegratorOutMin=[]  IntegratorOutMax=[]  FilterOutMin=[]  FilterOutMax=[]  SumI1OutMin=[]  SumI1OutMax=[]  SumI2OutMin=[]  SumI2OutMax=[]  SumI3OutMin=[]  SumI3OutMax=[]  SumI4OutMin=[]  SumI4OutMax=[]  SumDOutMin=[]  SumDOutMax=[]  DifferentiatorOutMin=[]  DifferentiatorOutMax=[]  FilterDiffOutCoefMin=[]  FilterDiffOutCoefMax=[]  ReciprocalOutMin=[]  ReciprocalOutMax=[]  SumDenOutMin=[]  SumDenOutMax=[]  SumNumOutMin=[]  SumNumOutMax=[]  DivideOutMin=[]  DivideOutMax=[]  IntegratorContinuousStateAttributes=''  IntegratorStateMustResolveToSignalObject=off  IntegratorRTWStateStorageClass=Auto  FilterContinuousStateAttributes=''  FilterStateMustResolveToSignalObject=off  FilterRTWStateStorageClass=Auto  ParallelPVariant=Passthrough  IdealPVariant=InternalParameters  IVariant=InternalParameters  DVariant=Disabled  IntegratorVariant=Continuous  SatVariant=Enabled  AWVariant=ContClampingIdeal  PCopyVariant=InternalParamsIdeal  TRVariant=Disabled  FdbkBlocksVariant=Forward  IdealPFdbkVariant=Disabled  SatFdbkVariant=Disabled  DerivativeFilterVariant=Disabled  NVariant=Disabled  NCopyVariant=Disabled_SignalSpec  FilterICVariant=Disabled  IntegratorICVariant=InternalICs  ExternalResetVariant=Disabled  TRSumVariant=Passthrough  SumFdbkVariant=Disabled  SumVariant=Sum_PI
  Product : Product
  Sum13 : Sum  Inputs=|+-
  Transfer Fcn (with initial states) : Subsystem  mask(Transfer Function with Initial States){N=[1], D=[timeconst 1], X0=0}
      mask prompts: N "Numerator:"; D "Denominator:"; X0 "Initial conditions:"
      mask help: Vector expressions for numerator, and denominator. Coefficients are in descending powers of s.
      mask init:
      | [A,B,C,Dd]=tf2ss(N,D);if (isempty(X0));[m,n]=size(A);X0=zeros(1,m); end;
      mask Help: Specify the initial states for the transfer function.  The state ordering is determined by the m-file tf2ss.  There is no unique mapping of the states in a transfer function to states in a state-space representation.  However, tf2ss will consistently use the same mapping for a given transfer function.
      mask Display: dpoly(N,D,'s')
  convective : Gain  Gain=s_conv  SaturateOnIntegerOverflow=on  OutDataTypeStr=Inherit: Same as input  ParamDataTypeStr=Inherit: Same as input
  maximal power : Constant  Value=max_power
  radiative : Gain  Gain=1-s_conv  SaturateOnIntegerOverflow=on  OutDataTypeStr=Inherit: Same as input  ParamDataTypeStr=Inherit: Same as input
  "[S]" : Outport  VectorParamsAs1DForOutWhenUnconnected=off
  "[HVAC]" : Outport  Port=2  VectorParamsAs1DForOutWhenUnconnected=off
  wires:
  Bus Creator1/1 -> "[HVAC]"/1
  Integrator/1 -> Bus Creator1/2  "heating energy"
  temperature setpoint/1 -> Sum13/1
  Bus Selector5/1 -> Sum13/2  "<Ts>"
  Product/1 -> Mux1/4, Integrator/1, Bus Creator1/1, radiative/1, convective/1  "heating power"
  "   "/1 -> Mux1/3
  radiative/1 -> Mux1/2
  temperature room/1 -> Bus Selector5/1
  maximal power/1 -> Product/2
  PID/1 -> Transfer Fcn (with initial states)/1(In1)
  convective/1 -> Mux1/1
  Mux1/1 -> "[S]"/1
  " "/1 -> Mux1/5
  Transfer Fcn (with initial states)/1(Out1) -> Product/1
  Sum13/1 -> PID/1
